simulink model "EsercitazioneEsame_LMI_sim"  (R2025b)
settings: Solver=VariableStepAuto  StartTime=0.0  StopTime=10.0  RelTol=1e-3
values from neighbouring files (symbols this model uses):
  A = double(subs(A_sym, [x; u], [x_star; u_star]))    [EsercitazioneEsame.m]
  B = [0; 0]    [Controllo_Avanzato_1.m]    (also in EsercitazioneEsame.m = double(subs(B_sym, [x; u], [x_star; u_star])))
  C = eye(2)    [Controllo_Avanzato_1.m]    (also in EsercitazioneEsame.m = eye(n))
  D = 0    [Controllo_Avanzato_1.m]    (also in EsercitazioneEsame.m = zeros(n, size(B, 2)))
  K = L/Q    [EsercitazioneEsame.m]
  N = inv(G_statico)    [EsercitazioneEsame.m]
  x0 = [1; 0]    [Controllo_Avanzato_1.m]    (also in EsercitazioneEsame.m = [0.3)
  x_ref = [h1_ref ... (first row only)    [EsercitazioneEsame.m]
settings Model: Creator=salvo  LastModifiedBy=salvo

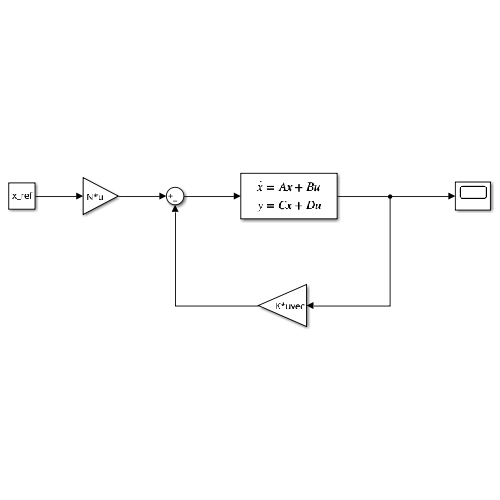
[thumbnail: Simulink's stored preview of the top-level diagram]
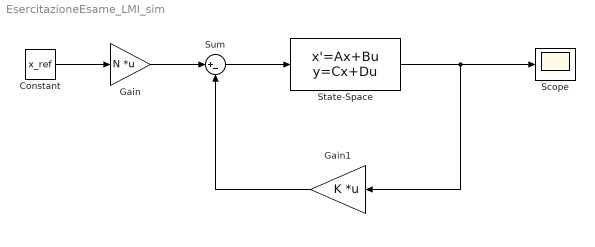
== system EsercitazioneEsame_LMI_sim ==
  Constant : Constant  Value=x_ref
  Gain : Gain  Gain=N  Multiplication=Matrix(K*u)
  Gain1 : Gain  Gain=K  Multiplication=Matrix(K*u) (u vector)
  Scope : Scope
      settings: ActiveDisplayYMinimum=-0.23670716257722413  ActiveDisplayYMaximum=0.84162188192947562
  State-Space : StateSpace  A=A  B=B  C=C  D=D  InitialCondition=x0
  Sum : Sum  Inputs=|+-
  wires:
  Sum/1 -> State-Space/1
  State-Space/1 -> Scope/1, Gain1/1
  Gain1/1 -> Sum/2
  Gain/1 -> Sum/1
  Constant/1 -> Gain/1
